simulink model "drillingRigMss"  (R2016a)
settings: Solver=VariableStepAuto  StartTime=0.0  StopTime=100  RelTol=1e-3
values from neighbouring files (symbols this model uses):
  EstimateFuelConsumption = 1    [initDrillingRigMSStoolbox.m]
  vNL0 = voltageNoQLoad*ones(engines,1)    [initDrillingRigMSStoolbox.m]
  wNL0 = 1./(1-Droop*.5)    [initDrillingRigMSStoolbox.m]
undefined symbols (not defined in the file or in its folder): magnitude, nr
undefined symbols (not defined in the file): generators
libraries: simulink x3, switchboard x1
settings Model: Creator=Elend  LastModifiedBy=torstebo
settings DataIOCC: LimitDataPoints=on  SaveFormat=Array  InspectSignalLogs=on
settings DebuggingCC: UnderspecifiedInitializationDetection=Classic  MergeDetectMultiDrivingBlocksExec=none  SolverPrmCheckMsg=warning  StateNameClashWarn=warning
settings HardwareCC: ProdBitPerPointer=32  ProdLargestAtomicFloat=None  ProdIntDivRoundTo=Undefined  ProdEndianess=Unspecified  ProdWordSize=32  ProdHWDeviceType=32-bit Generic
settings ModelReferenceCC: PropagateSignalLabelsOutOfModel=off
settings ConfigComp: CovModelRefEnable=Off

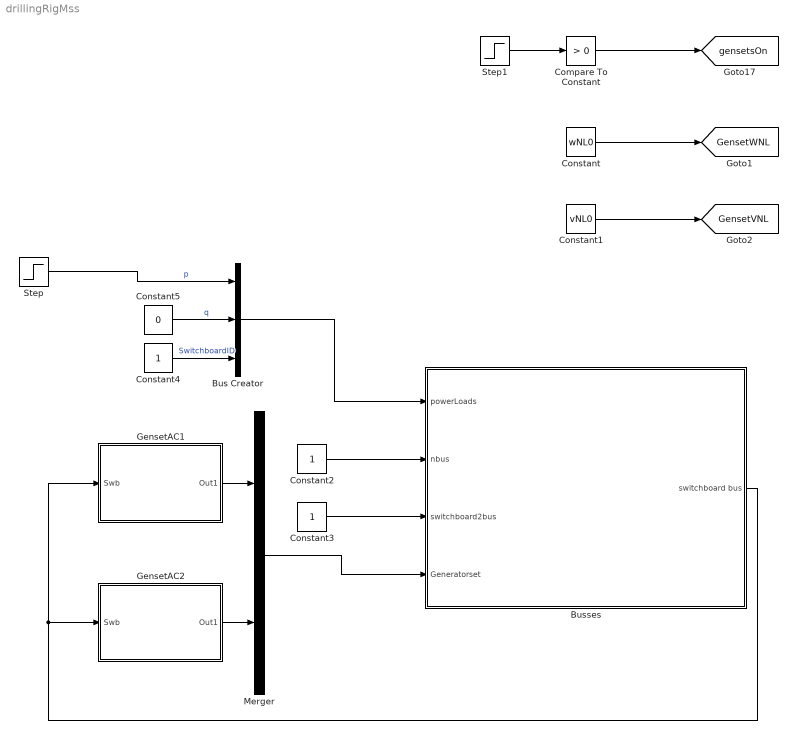
== system drillingRigMss ==
  Bus Creator : BusCreator  Inputs='p','q','SwitchboardID'  OutDataTypeStr=Bus: powerLoadsBus  NonVirtualBus=on
  Busses : Subsystem
      mask Display:
      | image(imread('figs/switchboard.jpg'))
      | port_label('input',1,'Power Loads')
      | port_label('input',2,'nbus')
      | port_label('input',3,'switchboard2bus')
      | port_label('input',4,'Generators')
      | port_label('output',1,'switchboard')
  Compare To Constant : simulink/Logic and Bit Operations/Compare To Constant  relop=>  const=0  OutDataTypeStr=boolean
  Constant : Constant  Value=wNL0
  Constant1 : Constant  Value=vNL0
  Constant2 : Constant
  Constant3 : Constant
  Constant4 : Constant
  Constant5 : Constant  Value=0
  GensetAC1 : Subsystem  Tag=GensetAC  mask{genset=generators(1), swbId=1}
      mask prompts: genset "Generator set data"; swbId "SwitchboardId"
      mask Display: image(imread('figs/generator.jpg'),'center')
  GensetAC2 : Subsystem  Tag=GensetAC  mask{genset=generators(2), swbId=1}
      mask prompts: genset "Generator set data"; swbId "SwitchboardId"
      mask Display: image(imread('figs/generator.jpg'),'center')
  Merger : Concatenate  Tag=FromGeneratorsetElectric/Merger
  Step : Step  Time=5  Before=1e6  After=2e6  SampleTime=0
  Step1 : Step  Time=50  Before=[1;1]  After=[1;0]  SampleTime=0
  tag scope: GensetVNL=global, GensetWNL=global, gensetsOn=global
  wires:
  Step1/1 -> Compare To Constant/1
  Compare To Constant/1 -> [gensetsOn]
  Constant/1 -> [GensetWNL]
  Constant1/1 -> [GensetVNL]
  Bus Creator/1 -> Busses/1(powerLoads)
  Constant3/1 -> Busses/3(switchboard2bus)
  Constant2/1 -> Busses/2(nbus)
  GensetAC2/1(Out1) -> Merger/2
  GensetAC1/1(Out1) -> Merger/1
  Merger/1 -> Busses/4(Generatorset)
  Step/1 -> Bus Creator/1  "p"
  Constant4/1 -> Bus Creator/3  "SwitchboardID"
  Constant5/1 -> Bus Creator/2  "q"
  Busses/1(switchboard bus) -> GensetAC2/1(Swb), GensetAC1/1(Swb)

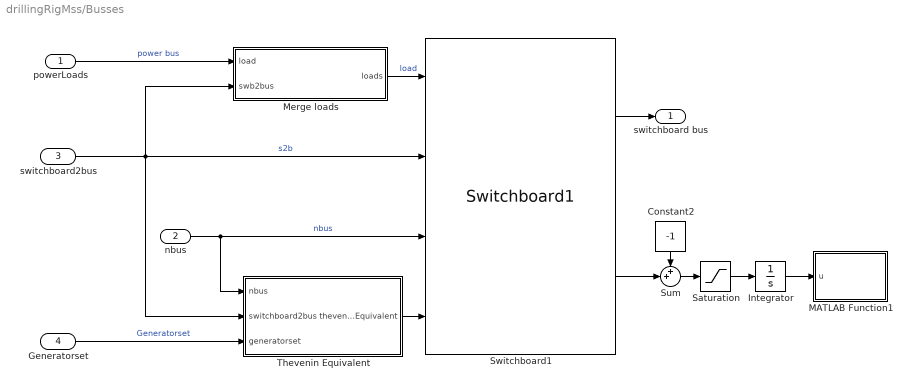
== system drillingRigMss/Busses ==
  powerLoads : Inport  OutDataTypeStr=Bus: powerLoadsBus
  nbus : Inport  Port=2
  switchboard2bus : Inport  Port=3
  Generatorset : Inport  Port=4
  Constant2 : Constant  Value=-1
  Integrator : Integrator
  MATLAB Function1 : MATLAB Function  TreatAsAtomicUnit=on
  Merge loads : MATLAB Function  TreatAsAtomicUnit=on
  Saturation : Saturate  UpperLimit=0  LowerLimit=-1
  Sum : Sum  Inputs=++|
  Switchboard1 : switchboard/Switchboard1
  Thevenin Equivalent : MATLAB Function  TreatAsAtomicUnit=on
  switchboard bus : Outport
  wires:
  Switchboard1/1 -> switchboard bus/1
  powerLoads/1 -> Merge loads/1(load)  "power bus"
  switchboard2bus/1 -> Thevenin Equivalent/2(switchboard2bus), Merge loads/2(swb2bus), Switchboard1/2  "s2b"
  Generatorset/1 -> Thevenin Equivalent/3(generatorset)  "Generatorset"
  Integrator/1 -> MATLAB Function1/1(u)
  Constant2/1 -> Sum/1
  Sum/1 -> Saturation/1
  Switchboard1/2 -> Sum/2
  nbus/1 -> Thevenin Equivalent/1(nbus), Switchboard1/3  "nbus"
  Merge loads/1(loads) -> Switchboard1/1  "load"
  Thevenin Equivalent/1(theveninEquivalent) -> Switchboard1/4
  Saturation/1 -> Integrator/1

== system drillingRigMss/GensetAC1 ==
  Swb : Inport
  Constant4 : Constant  Value=genset.ID  OutDataTypeStr=Inherit: Inherit via back propagation
  Genset : Subsystem
  Goto Tag Visibility : GotoTagVisibility  GotoTag=connected
  Selector : Selector  IndexOptions=Index vector (port)  Indices=[nr]  OutputSizes=1
  Out1 : Outport
  tag scope: connected=scoped
  wires:
  Genset/1(TheveninBus) -> Out1/1
  Constant4/1 -> Selector/2
  [gensetsOn] -> Selector/1  "Connected"
  Selector/1 -> [connected]  "Connected"
  Swb/1 -> Genset/1(Switchboard)

== system drillingRigMss/GensetAC2 ==
  Swb : Inport
  Constant4 : Constant  Value=genset.ID  OutDataTypeStr=Inherit: Inherit via back propagation
  Genset : Subsystem
  Goto Tag Visibility : GotoTagVisibility  GotoTag=connected
  Selector : Selector  IndexOptions=Index vector (port)  Indices=[nr]  OutputSizes=1
  Out1 : Outport
  tag scope: connected=scoped
  wires:
  Genset/1(TheveninBus) -> Out1/1
  Constant4/1 -> Selector/2
  [gensetsOn] -> Selector/1  "Connected"
  Selector/1 -> [connected]  "Connected"
  Swb/1 -> Genset/1(Switchboard)

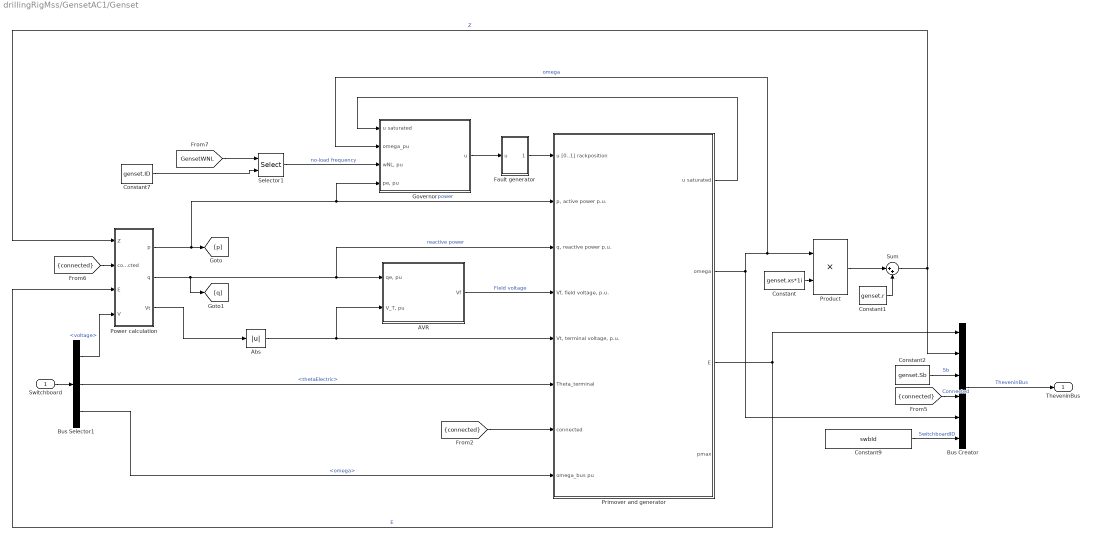
== system drillingRigMss/GensetAC1/Genset ==
  Switchboard : Inport
  AVR : Subsystem
  Abs : Abs
  Bus Creator : BusCreator  Inputs='E','Z','Sb','Connected','omega','SwitchboardID'  OutDataTypeStr=Bus: TheveninBus  NonVirtualBus=on
  Bus Selector1 : BusSelector  OutputSignals=voltage,thetaElectric,omega
  Constant : Constant  Value=genset.xs*1i
  Constant1 : Constant  Value=genset.r
  Constant2 : Constant  Value=genset.Sb
  Constant7 : Constant  Value=genset.ID  OutDataTypeStr=Inherit: Inherit via back propagation
  Constant9 : Constant  Value=swbId  OutDataTypeStr=Inherit: Inherit via back propagation
  Fault generator : Subsystem
  Governor : Subsystem
  Power calculation : MATLAB Function  TreatAsAtomicUnit=on
  Primover and generator : Subsystem
  Product : Product
  Selector1 : Selector  IndexOptions=Index vector (port)  Indices=[nr]  OutputSizes=1
  Sum : Sum  Inputs=|++
  TheveninBus : Outport
  wires:
  Constant7/1 -> Selector1/2
  Constant2/1 -> Bus Creator/3  "Sb"
  Bus Creator/1 -> TheveninBus/1  "TheveninBus"
  Sum/1 -> Bus Creator/2, Power calculation/1(Z)  "Z"
  Constant1/1 -> Sum/2
  Product/1 -> Sum/1
  Constant/1 -> Product/2
  Abs/1 -> AVR/2("V_T, pu"), Primover and generator/5("Vt, terminal voltage, p.u.")
  Power calculation/2(q) -> [q], AVR/1("qe, pu"), Primover and generator/3("q, reactive power p.u.")  "reactive power"
  Power calculation/1(p) -> [p], Governor/4("pe, pu"), Primover and generator/2("p, active power p.u.")  "power"
  [GensetWNL] -> Selector1/1
  Primover and generator/3(E) -> Bus Creator/1, Power calculation/3(E)  "E"
  Primover and generator/2(omega) -> Product/1, Governor/2(omega_pu), Bus Creator/5  "omega"
  Primover and generator/1(u saturated) -> Governor/1(u saturated)
  AVR/1(Vf) -> Primover and generator/4("Vf, field voltage, p.u.")  "Field voltage"
  Selector1/1 -> Governor/3("wNL, pu")  "no-load frequency"
  Bus Selector1/1 -> Power calculation/4(V)  "<voltage>"
  [connected] -> Primover and generator/7(connected)
  [connected] -> Power calculation/2(connected)
  [connected] -> Bus Creator/4  "Connected"
  Power calculation/3(Vt) -> Abs/1
  Bus Selector1/3 -> Primover and generator/8(omega_bus pu)  "<omega>"
  Switchboard/1 -> Bus Selector1/1
  Constant9/1 -> Bus Creator/6  "SwitchboardID"
  Bus Selector1/2 -> Primover and generator/6(Theta_terminal)  "<thetaElectric>"
  Governor/1(u) -> Fault generator/1(u)
  Fault generator/1(uOut) -> Primover and generator/1(u [0..1] rackposition)

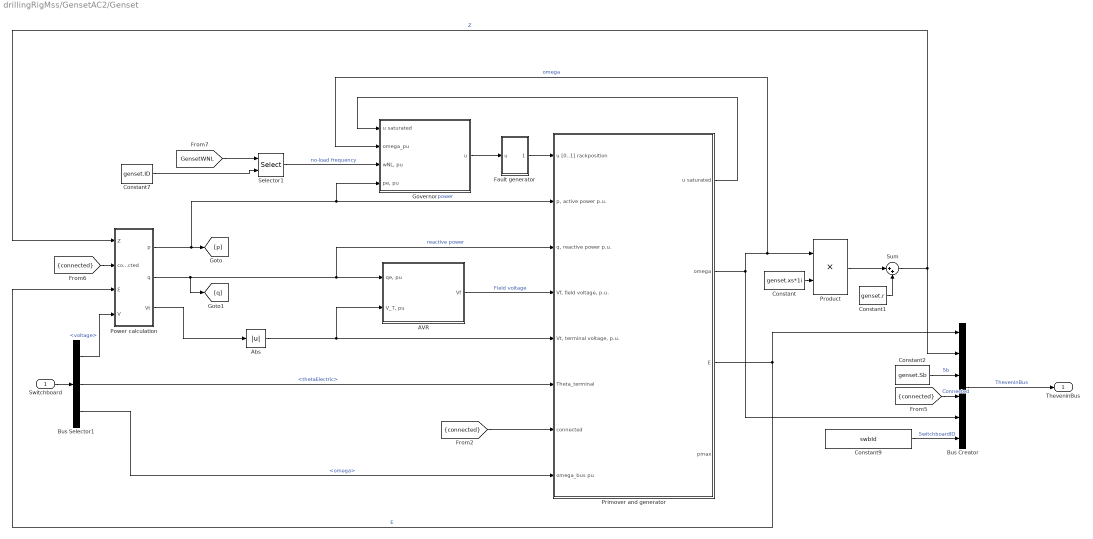
== system drillingRigMss/GensetAC2/Genset ==
  Switchboard : Inport
  AVR : Subsystem
  Abs : Abs
  Bus Creator : BusCreator  Inputs='E','Z','Sb','Connected','omega','SwitchboardID'  OutDataTypeStr=Bus: TheveninBus  NonVirtualBus=on
  Bus Selector1 : BusSelector  OutputSignals=voltage,thetaElectric,omega
  Constant : Constant  Value=genset.xs*1i
  Constant1 : Constant  Value=genset.r
  Constant2 : Constant  Value=genset.Sb
  Constant7 : Constant  Value=genset.ID  OutDataTypeStr=Inherit: Inherit via back propagation
  Constant9 : Constant  Value=swbId  OutDataTypeStr=Inherit: Inherit via back propagation
  Fault generator : Subsystem
  Governor : Subsystem
  Power calculation : MATLAB Function  TreatAsAtomicUnit=on
  Primover and generator : Subsystem
  Product : Product
  Selector1 : Selector  IndexOptions=Index vector (port)  Indices=[nr]  OutputSizes=1
  Sum : Sum  Inputs=|++
  TheveninBus : Outport
  wires:
  Constant7/1 -> Selector1/2
  Constant2/1 -> Bus Creator/3  "Sb"
  Bus Creator/1 -> TheveninBus/1  "TheveninBus"
  Sum/1 -> Bus Creator/2, Power calculation/1(Z)  "Z"
  Constant1/1 -> Sum/2
  Product/1 -> Sum/1
  Constant/1 -> Product/2
  Abs/1 -> AVR/2("V_T, pu"), Primover and generator/5("Vt, terminal voltage, p.u.")
  Power calculation/2(q) -> [q], AVR/1("qe, pu"), Primover and generator/3("q, reactive power p.u.")  "reactive power"
  Power calculation/1(p) -> [p], Governor/4("pe, pu"), Primover and generator/2("p, active power p.u.")  "power"
  [GensetWNL] -> Selector1/1
  Primover and generator/3(E) -> Bus Creator/1, Power calculation/3(E)  "E"
  Primover and generator/2(omega) -> Product/1, Governor/2(omega_pu), Bus Creator/5  "omega"
  Primover and generator/1(u saturated) -> Governor/1(u saturated)
  AVR/1(Vf) -> Primover and generator/4("Vf, field voltage, p.u.")  "Field voltage"
  Selector1/1 -> Governor/3("wNL, pu")  "no-load frequency"
  Bus Selector1/1 -> Power calculation/4(V)  "<voltage>"
  [connected] -> Primover and generator/7(connected)
  [connected] -> Power calculation/2(connected)
  [connected] -> Bus Creator/4  "Connected"
  Power calculation/3(Vt) -> Abs/1
  Bus Selector1/3 -> Primover and generator/8(omega_bus pu)  "<omega>"
  Switchboard/1 -> Bus Selector1/1
  Constant9/1 -> Bus Creator/6  "SwitchboardID"
  Bus Selector1/2 -> Primover and generator/6(Theta_terminal)  "<thetaElectric>"
  Governor/1(u) -> Fault generator/1(u)
  Fault generator/1(uOut) -> Primover and generator/1(u [0..1] rackposition)

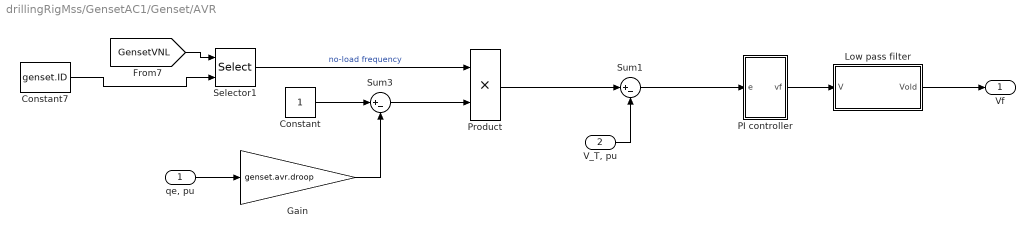
== system drillingRigMss/GensetAC1/Genset/AVR ==
  "qe, pu" : Inport
  "V_T, pu" : Inport  Port=2
  Constant : Constant
  Constant7 : Constant  Value=genset.ID  OutDataTypeStr=Inherit: Inherit via back propagation
  Gain : Gain  Gain=genset.avr.droop
  Low pass filter : Subsystem
  PI controller : Subsystem
  Product : Product  RndMeth=Zero
  Selector1 : Selector  IndexOptions=Index vector (port)  Indices=[nr]  OutputSizes=1
  Sum1 : Sum  Inputs=|+-
  Sum3 : Sum  Inputs=|+-
  Vf : Outport
  wires:
  Low pass filter/1(Vold) -> Vf/1
  Product/1 -> Sum1/1
  Sum3/1 -> Product/2
  Gain/1 -> Sum3/2
  Constant/1 -> Sum3/1
  "V_T, pu"/1 -> Sum1/2
  "qe, pu"/1 -> Gain/1
  Sum1/1 -> PI controller/1(e)
  PI controller/1(vf) -> Low pass filter/1(V)
  Constant7/1 -> Selector1/2
  [GensetVNL] -> Selector1/1
  Selector1/1 -> Product/1  "no-load frequency"

== system drillingRigMss/GensetAC1/Genset/Fault generator ==
  u : Inport
  Constant4 : Constant  Value=genset.fixThrottle
  Step : Step  Time=genset.fixThrottleTime  SampleTime=0
  Switch : Switch  Criteria=u2 > Threshold
  uOut : Outport
  wires:
  Switch/1 -> uOut/1
  u/1 -> Switch/3
  Constant4/1 -> Switch/1
  Step/1 -> Switch/2

== system drillingRigMss/GensetAC1/Genset/Governor ==
  u saturated : Inport
  omega_pu : Inport  Port=2
  "wNL, pu" : Inport  Port=3
  "pe, pu" : Inport  Port=4
  Constant : Constant
  Gain : Gain  Gain=genset.governor.droop
  PID controller : Subsystem
  Product : Product  RndMeth=Zero
  Sum : Sum  Inputs=|+-
  Sum1 : Sum  Inputs=|+-
  u : Outport
  wires:
  omega_pu/1 -> PID controller/2(omega_pu), Sum/2
  "pe, pu"/1 -> Gain/1
  u saturated/1 -> PID controller/3(u saturated)
  Sum1/1 -> Product/2
  Constant/1 -> Sum1/1
  "wNL, pu"/1 -> Product/1
  Product/1 -> Sum/1
  Sum/1 -> PID controller/1(e)
  Gain/1 -> Sum1/2
  PID controller/1(u) -> u/1  "u"

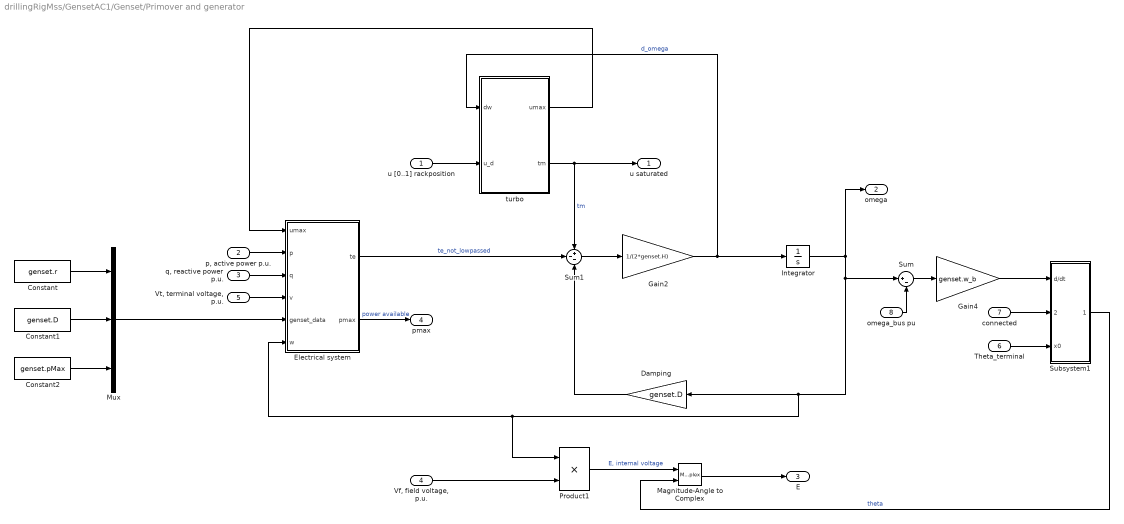
== system drillingRigMss/GensetAC1/Genset/Primover and generator ==
  u [0..1] rackposition : Inport
  "p, active power p.u." : Inport  Port=2
  "q, reactive power p.u." : Inport  Port=3
  "Vf, field voltage, p.u." : Inport  Port=4
  "Vt, terminal voltage, p.u." : Inport  Port=5
  Theta_terminal : Inport  Port=6
  connected : Inport  Port=7
  omega_bus pu : Inport  Port=8
  Constant : Constant  Value=genset.r
  Constant1 : Constant  Value=genset.D
  Constant2 : Constant  Value=genset.pMax
  Damping : Gain  Gain=genset.D
  Electrical system : MATLAB Function  TreatAsAtomicUnit=on
  Gain2 : Gain  Gain=1/(2*genset.H)
  Gain4 : Gain  Gain=genset.w_b
  Integrator : Integrator  InitialCondition=genset.omega0
  Magnitude-Angle to Complex : MagnitudeAngleToComplex
  Mux : Mux  Inputs=3
  Product1 : Product  Inputs=**  RndMeth=Zero
  Subsystem1 : Subsystem
  Sum : Sum  Inputs=|+-
  Sum1 : Sum  Inputs=+--
  turbo : Subsystem
  u saturated : Outport
  omega : Outport  Port=2
  E : Outport  Port=3
  pmax : Outport  Port=4
  wires:
  Mux/1 -> Electrical system/5(genset_data)
  Constant2/1 -> Mux/3
  Constant1/1 -> Mux/2
  Constant/1 -> Mux/1
  Magnitude-Angle to Complex/1 -> E/1
  Electrical system/2(pmax) -> pmax/1  "power available"
  turbo/1(umax) -> Electrical system/1(umax)
  Theta_terminal/1 -> Subsystem1/3(x0)
  Integrator/1 -> omega/1, Electrical system/6(w), Product1/1, Damping/1, Sum/1
  connected/1 -> Subsystem1/2(reset)
  Damping/1 -> Sum1/3
  "q, reactive power p.u."/1 -> Electrical system/3(q)
  "Vt, terminal voltage, p.u."/1 -> Electrical system/4(v)
  Electrical system/1(te) -> Sum1/2  "te_not_lowpassed"
  "p, active power p.u."/1 -> Electrical system/2(p)
  "Vf, field voltage, p.u."/1 -> Product1/2
  Gain2/1 -> Integrator/1, turbo/1(dw)  "d_omega"
  Sum1/1 -> Gain2/1
  Gain4/1 -> Subsystem1/1(d/dt)
  Subsystem1/1(Out1) -> Magnitude-Angle to Complex/2  "theta"
  Product1/1 -> Magnitude-Angle to Complex/1  "E, internal voltage"
  turbo/2(tm) -> Sum1/1, u saturated/1  "tm"
  u [0..1] rackposition/1 -> turbo/2(u_d)
  Sum/1 -> Gain4/1
  omega_bus pu/1 -> Sum/2

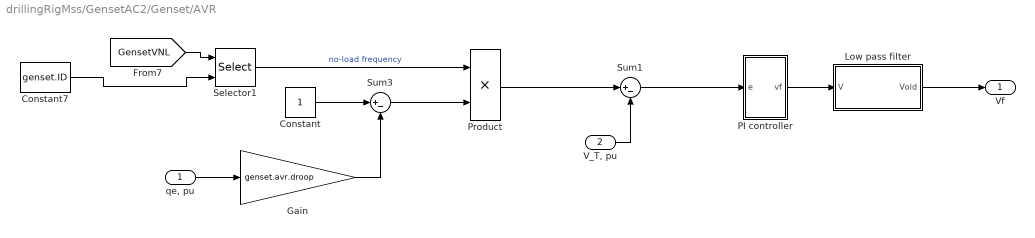
== system drillingRigMss/GensetAC2/Genset/AVR ==
  "qe, pu" : Inport
  "V_T, pu" : Inport  Port=2
  Constant : Constant
  Constant7 : Constant  Value=genset.ID  OutDataTypeStr=Inherit: Inherit via back propagation
  Gain : Gain  Gain=genset.avr.droop
  Low pass filter : Subsystem
  PI controller : Subsystem
  Product : Product  RndMeth=Zero
  Selector1 : Selector  IndexOptions=Index vector (port)  Indices=[nr]  OutputSizes=1
  Sum1 : Sum  Inputs=|+-
  Sum3 : Sum  Inputs=|+-
  Vf : Outport
  wires:
  Low pass filter/1(Vold) -> Vf/1
  Product/1 -> Sum1/1
  Sum3/1 -> Product/2
  Gain/1 -> Sum3/2
  Constant/1 -> Sum3/1
  "V_T, pu"/1 -> Sum1/2
  "qe, pu"/1 -> Gain/1
  Sum1/1 -> PI controller/1(e)
  PI controller/1(vf) -> Low pass filter/1(V)
  Constant7/1 -> Selector1/2
  [GensetVNL] -> Selector1/1
  Selector1/1 -> Product/1  "no-load frequency"

== system drillingRigMss/GensetAC2/Genset/Fault generator ==
  u : Inport
  Constant4 : Constant  Value=genset.fixThrottle
  Step : Step  Time=genset.fixThrottleTime  SampleTime=0
  Switch : Switch  Criteria=u2 > Threshold
  uOut : Outport
  wires:
  Switch/1 -> uOut/1
  u/1 -> Switch/3
  Constant4/1 -> Switch/1
  Step/1 -> Switch/2

== system drillingRigMss/GensetAC2/Genset/Governor ==
  u saturated : Inport
  omega_pu : Inport  Port=2
  "wNL, pu" : Inport  Port=3
  "pe, pu" : Inport  Port=4
  Constant : Constant
  Gain : Gain  Gain=genset.governor.droop
  PID controller : Subsystem
  Product : Product  RndMeth=Zero
  Sum : Sum  Inputs=|+-
  Sum1 : Sum  Inputs=|+-
  u : Outport
  wires:
  omega_pu/1 -> PID controller/2(omega_pu), Sum/2
  "pe, pu"/1 -> Gain/1
  u saturated/1 -> PID controller/3(u saturated)
  Sum1/1 -> Product/2
  Constant/1 -> Sum1/1
  "wNL, pu"/1 -> Product/1
  Product/1 -> Sum/1
  Sum/1 -> PID controller/1(e)
  Gain/1 -> Sum1/2
  PID controller/1(u) -> u/1  "u"

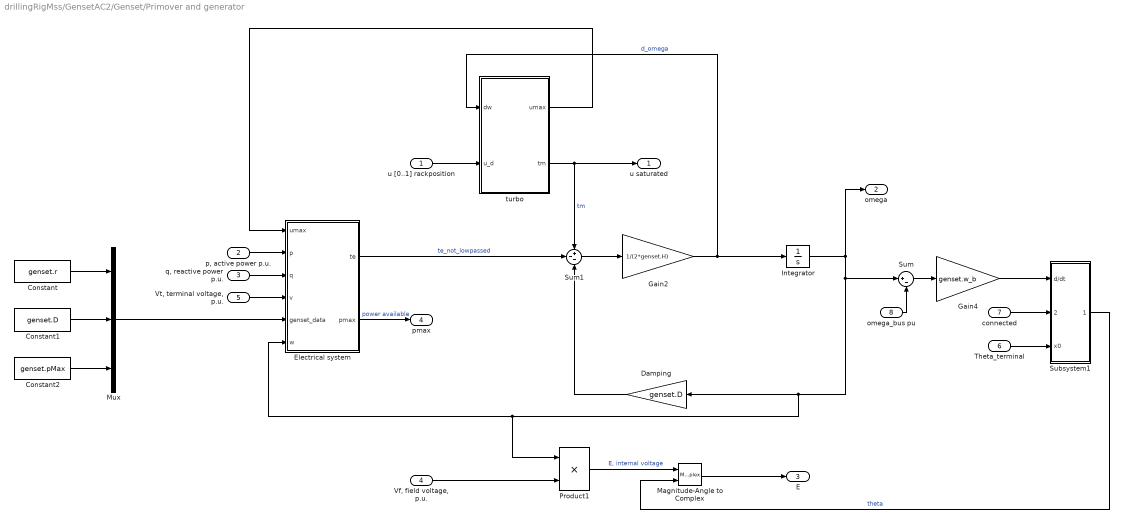
== system drillingRigMss/GensetAC2/Genset/Primover and generator ==
  u [0..1] rackposition : Inport
  "p, active power p.u." : Inport  Port=2
  "q, reactive power p.u." : Inport  Port=3
  "Vf, field voltage, p.u." : Inport  Port=4
  "Vt, terminal voltage, p.u." : Inport  Port=5
  Theta_terminal : Inport  Port=6
  connected : Inport  Port=7
  omega_bus pu : Inport  Port=8
  Constant : Constant  Value=genset.r
  Constant1 : Constant  Value=genset.D
  Constant2 : Constant  Value=genset.pMax
  Damping : Gain  Gain=genset.D
  Electrical system : MATLAB Function  TreatAsAtomicUnit=on
  Gain2 : Gain  Gain=1/(2*genset.H)
  Gain4 : Gain  Gain=genset.w_b
  Integrator : Integrator  InitialCondition=genset.omega0
  Magnitude-Angle to Complex : MagnitudeAngleToComplex
  Mux : Mux  Inputs=3
  Product1 : Product  Inputs=**  RndMeth=Zero
  Subsystem1 : Subsystem
  Sum : Sum  Inputs=|+-
  Sum1 : Sum  Inputs=+--
  turbo : Subsystem
  u saturated : Outport
  omega : Outport  Port=2
  E : Outport  Port=3
  pmax : Outport  Port=4
  wires:
  Mux/1 -> Electrical system/5(genset_data)
  Constant2/1 -> Mux/3
  Constant1/1 -> Mux/2
  Constant/1 -> Mux/1
  Magnitude-Angle to Complex/1 -> E/1
  Electrical system/2(pmax) -> pmax/1  "power available"
  turbo/1(umax) -> Electrical system/1(umax)
  Theta_terminal/1 -> Subsystem1/3(x0)
  Integrator/1 -> omega/1, Electrical system/6(w), Product1/1, Damping/1, Sum/1
  connected/1 -> Subsystem1/2(reset)
  Damping/1 -> Sum1/3
  "q, reactive power p.u."/1 -> Electrical system/3(q)
  "Vt, terminal voltage, p.u."/1 -> Electrical system/4(v)
  Electrical system/1(te) -> Sum1/2  "te_not_lowpassed"
  "p, active power p.u."/1 -> Electrical system/2(p)
  "Vf, field voltage, p.u."/1 -> Product1/2
  Gain2/1 -> Integrator/1, turbo/1(dw)  "d_omega"
  Sum1/1 -> Gain2/1
  Gain4/1 -> Subsystem1/1(d/dt)
  Subsystem1/1(Out1) -> Magnitude-Angle to Complex/2  "theta"
  Product1/1 -> Magnitude-Angle to Complex/1  "E, internal voltage"
  turbo/2(tm) -> Sum1/1, u saturated/1  "tm"
  u [0..1] rackposition/1 -> turbo/2(u_d)
  Sum/1 -> Gain4/1
  omega_bus pu/1 -> Sum/2

== system drillingRigMss/GensetAC1/Genset/AVR/Low pass filter ==
  V : Inport
  Gain : Gain  Gain=1/genset.avr.T
  Integrator : Integrator  InitialCondition=genset.avr.v0
  Sum : Sum  Inputs=|+-
  Vold : Outport
  wires:
  Gain/1 -> Integrator/1
  Sum/1 -> Gain/1
  V/1 -> Sum/1
  Integrator/1 -> Sum/2, Vold/1

== system drillingRigMss/GensetAC1/Genset/AVR/PI controller ==
  e : Inport
  Gain : Gain  Gain=genset.avr.ki
  Gain1 : Gain  Gain=genset.avr.kp
  Integrator : Integrator  DisableCoverage=on  InitialCondition=genset.avr.v0
  Saturation : Saturate  UpperLimit=genset.avr.maxFieldVoltage  LowerLimit=genset.avr.minFieldVoltage  LinearizeAsGain=off  OutMin=genset.avr.minFieldVoltage  OutMax=genset.avr.maxFieldVoltage  OutDataTypeStr=Inherit: Inherit via back propagation
  Sum : Sum  Inputs=+|+
  vf : Outport
  wires:
  Gain/1 -> Integrator/1
  Gain1/1 -> Sum/1
  Integrator/1 -> Sum/2
  e/1 -> Gain1/1, Gain/1
  Sum/1 -> Saturation/1
  Saturation/1 -> vf/1

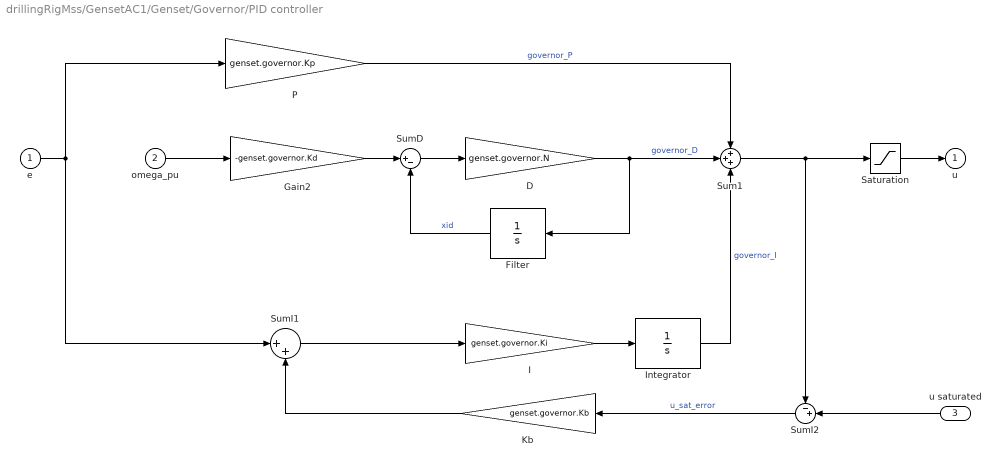
== system drillingRigMss/GensetAC1/Genset/Governor/PID controller ==
  e : Inport  PortDimensions=1
  omega_pu : Inport  Port=2  PortDimensions=1
  u saturated : Inport  Port=3  PortDimensions=1
  D : Gain  DisableCoverage=on  Gain=genset.governor.N
  Filter : Integrator  DisableCoverage=on  InitialCondition=-genset.omega0*genset.governor.Kd
  Gain2 : Gain  Gain=-genset.governor.Kd
  I : Gain  Gain=genset.governor.Ki
  Integrator : Integrator  DisableCoverage=on  InitialCondition=genset.u0
  Kb : Gain  DisableCoverage=on  Gain=genset.governor.Kb  ParamDataTypeStr=Inherit: Inherit from 'Gain'
  P : Gain  Gain=genset.governor.Kp
  Saturation : Saturate  UpperLimit=genset.uMax  LowerLimit=genset.uMin  LinearizeAsGain=off  OutMin=genset.uMin  OutMax=genset.uMax  OutDataTypeStr=Inherit: Inherit via back propagation
  Sum1 : Sum  Inputs=+++
  SumD : Sum  DisableCoverage=on  Inputs=|+-
  SumI1 : Sum  DisableCoverage=on  Inputs=|++
  SumI2 : Sum  DisableCoverage=on  Inputs=-+|
  u : Outport  PortDimensions=1  InitialOutput=0
  wires:
  I/1 -> Integrator/1
  SumI1/1 -> I/1
  u saturated/1 -> SumI2/2
  Kb/1 -> SumI1/2
  SumI2/1 -> Kb/1  "u_sat_error"
  Sum1/1 -> SumI2/1, Saturation/1
  Gain2/1 -> SumD/1
  SumD/1 -> D/1
  Filter/1 -> SumD/2  "xid"
  Saturation/1 -> u/1
  P/1 -> Sum1/1  "governor_P"
  e/1 -> SumI1/1, P/1
  omega_pu/1 -> Gain2/1
  D/1 -> Filter/1, Sum1/2  "governor_D"
  Integrator/1 -> Sum1/3  "governor_I"

== system drillingRigMss/GensetAC1/Genset/Primover and generator/Subsystem1 ==
  d/dt : Inport
  reset : Inport  Port=2
  x0 : Inport  Port=3
  Gain : Gain  Gain=1000
  Integrator : Integrator  InitialCondition=genset.theta0
  MATLAB Function : MATLAB Function  TreatAsAtomicUnit=on
  Sum : Sum  Inputs=-|+
  Switch : Switch  Threshold=1
  Out1 : Outport
  wires:
  Switch/1 -> Integrator/1
  d/dt/1 -> Switch/1
  MATLAB Function/1(y) -> Gain/1
  Gain/1 -> Switch/3
  Sum/1 -> MATLAB Function/1(u)
  x0/1 -> Sum/2
  reset/1 -> Switch/2
  Integrator/1 -> Sum/1, Out1/1

== system drillingRigMss/GensetAC1/Genset/Primover and generator/turbo ==
  dw : Inport
  u_d : Inport  Port=2
  Constant : Constant  Value=EstimateFuelConsumption
  Subsystem : Subsystem
  dead-band rate limiter : Subsystem  mask(Rate limiter for diesel engines){umax=genset.uMax, umin=genset.uMin}
      mask prompts: umax "Static maximum torque"; umin "Static minimum torque"
      mask help:
      | Allows the input to change within a delta limit, however if the input
      | changes more than this range will the input be saturated by a rate limiter.
  umax : Outport
  tm : Outport  Port=2
  wires:
  dead-band rate limiter/1(u_max) -> umax/1
  u_d/1 -> dead-band rate limiter/1(u_d)
  dead-band rate limiter/2(u_saturated) -> Subsystem/2(tm), tm/1  "tm"
  dw/1 -> Subsystem/1(dw)
  Constant/1 -> Subsystem/Enable

== system drillingRigMss/GensetAC2/Genset/AVR/Low pass filter ==
  V : Inport
  Gain : Gain  Gain=1/genset.avr.T
  Integrator : Integrator  InitialCondition=genset.avr.v0
  Sum : Sum  Inputs=|+-
  Vold : Outport
  wires:
  Gain/1 -> Integrator/1
  Sum/1 -> Gain/1
  V/1 -> Sum/1
  Integrator/1 -> Sum/2, Vold/1

== system drillingRigMss/GensetAC2/Genset/AVR/PI controller ==
  e : Inport
  Gain : Gain  Gain=genset.avr.ki
  Gain1 : Gain  Gain=genset.avr.kp
  Integrator : Integrator  DisableCoverage=on  InitialCondition=genset.avr.v0
  Saturation : Saturate  UpperLimit=genset.avr.maxFieldVoltage  LowerLimit=genset.avr.minFieldVoltage  LinearizeAsGain=off  OutMin=genset.avr.minFieldVoltage  OutMax=genset.avr.maxFieldVoltage  OutDataTypeStr=Inherit: Inherit via back propagation
  Sum : Sum  Inputs=+|+
  vf : Outport
  wires:
  Gain/1 -> Integrator/1
  Gain1/1 -> Sum/1
  Integrator/1 -> Sum/2
  e/1 -> Gain1/1, Gain/1
  Sum/1 -> Saturation/1
  Saturation/1 -> vf/1

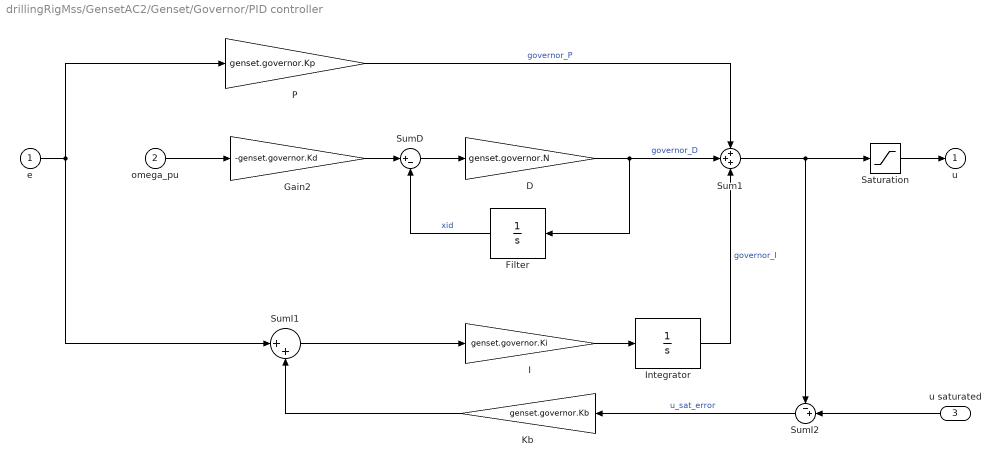
== system drillingRigMss/GensetAC2/Genset/Governor/PID controller ==
  e : Inport  PortDimensions=1
  omega_pu : Inport  Port=2  PortDimensions=1
  u saturated : Inport  Port=3  PortDimensions=1
  D : Gain  DisableCoverage=on  Gain=genset.governor.N
  Filter : Integrator  DisableCoverage=on  InitialCondition=-genset.omega0*genset.governor.Kd
  Gain2 : Gain  Gain=-genset.governor.Kd
  I : Gain  Gain=genset.governor.Ki
  Integrator : Integrator  DisableCoverage=on  InitialCondition=genset.u0
  Kb : Gain  DisableCoverage=on  Gain=genset.governor.Kb  ParamDataTypeStr=Inherit: Inherit from 'Gain'
  P : Gain  Gain=genset.governor.Kp
  Saturation : Saturate  UpperLimit=genset.uMax  LowerLimit=genset.uMin  LinearizeAsGain=off  OutMin=genset.uMin  OutMax=genset.uMax  OutDataTypeStr=Inherit: Inherit via back propagation
  Sum1 : Sum  Inputs=+++
  SumD : Sum  DisableCoverage=on  Inputs=|+-
  SumI1 : Sum  DisableCoverage=on  Inputs=|++
  SumI2 : Sum  DisableCoverage=on  Inputs=-+|
  u : Outport  PortDimensions=1  InitialOutput=0
  wires:
  I/1 -> Integrator/1
  SumI1/1 -> I/1
  u saturated/1 -> SumI2/2
  Kb/1 -> SumI1/2
  SumI2/1 -> Kb/1  "u_sat_error"
  Sum1/1 -> SumI2/1, Saturation/1
  Gain2/1 -> SumD/1
  SumD/1 -> D/1
  Filter/1 -> SumD/2  "xid"
  Saturation/1 -> u/1
  P/1 -> Sum1/1  "governor_P"
  e/1 -> SumI1/1, P/1
  omega_pu/1 -> Gain2/1
  D/1 -> Filter/1, Sum1/2  "governor_D"
  Integrator/1 -> Sum1/3  "governor_I"

== system drillingRigMss/GensetAC2/Genset/Primover and generator/Subsystem1 ==
  d/dt : Inport
  reset : Inport  Port=2
  x0 : Inport  Port=3
  Gain : Gain  Gain=1000
  Integrator : Integrator  InitialCondition=genset.theta0
  MATLAB Function : MATLAB Function  TreatAsAtomicUnit=on
  Sum : Sum  Inputs=-|+
  Switch : Switch  Threshold=1
  Out1 : Outport
  wires:
  Switch/1 -> Integrator/1
  d/dt/1 -> Switch/1
  MATLAB Function/1(y) -> Gain/1
  Gain/1 -> Switch/3
  Sum/1 -> MATLAB Function/1(u)
  x0/1 -> Sum/2
  reset/1 -> Switch/2
  Integrator/1 -> Sum/1, Out1/1

== system drillingRigMss/GensetAC2/Genset/Primover and generator/turbo ==
  dw : Inport
  u_d : Inport  Port=2
  Constant : Constant  Value=EstimateFuelConsumption
  Subsystem : Subsystem
  dead-band rate limiter : Subsystem  mask(Rate limiter for diesel engines){umax=genset.uMax, umin=genset.uMin}
      mask prompts: umax "Static maximum torque"; umin "Static minimum torque"
      mask help:
      | Allows the input to change within a delta limit, however if the input
      | changes more than this range will the input be saturated by a rate limiter.
  umax : Outport
  tm : Outport  Port=2
  wires:
  dead-band rate limiter/1(u_max) -> umax/1
  u_d/1 -> dead-band rate limiter/1(u_d)
  dead-band rate limiter/2(u_saturated) -> Subsystem/2(tm), tm/1  "tm"
  dw/1 -> Subsystem/1(dw)
  Constant/1 -> Subsystem/Enable

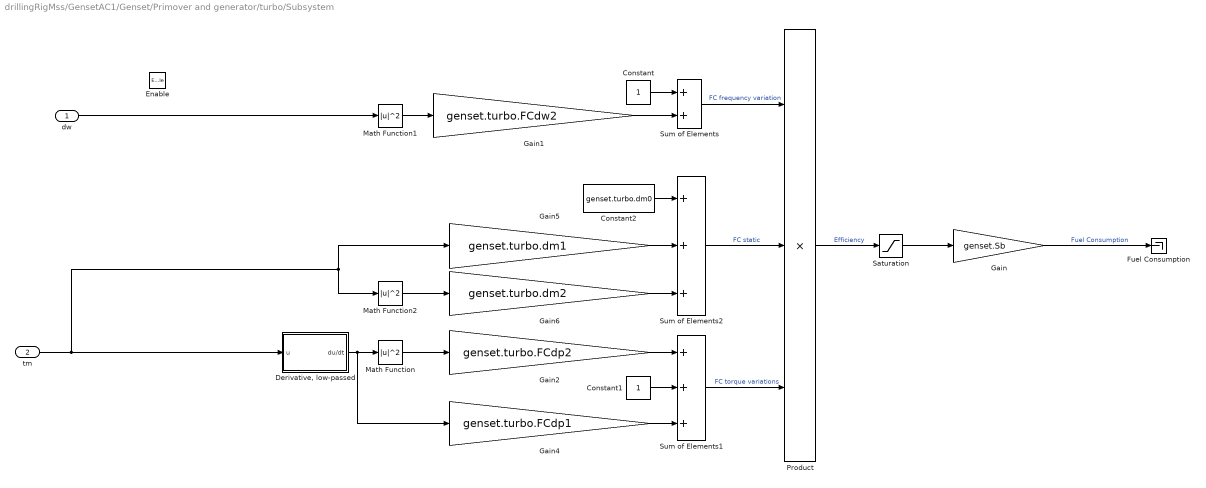
== system drillingRigMss/GensetAC1/Genset/Primover and generator/turbo/Subsystem ==
  dw : Inport
  tm : Inport  Port=2
  Enable : EnablePort
  Constant : Constant
  Constant1 : Constant
  Constant2 : Constant  Value=genset.turbo.dm0
  "Derivative, low-passed" : Subsystem
      settings: MinAlgLoopOccurrences=on
  Fuel Consumption : Terminator
  Gain : Gain  Gain=genset.Sb
  Gain1 : Gain  Gain=genset.turbo.FCdw2
  Gain2 : Gain  Gain=genset.turbo.FCdp2
  Gain4 : Gain  Gain=genset.turbo.FCdp1
  Gain5 : Gain  Gain=genset.turbo.dm1
  Gain6 : Gain  Gain=genset.turbo.dm2
  Math Function : Math  Operator=magnitude^2  SaturateOnIntegerOverflow=on
  Math Function1 : Math  Operator=magnitude^2  SaturateOnIntegerOverflow=on
  Math Function2 : Math  Operator=magnitude^2  SaturateOnIntegerOverflow=on
  Product : Product  Inputs=3  RndMeth=Zero
  Saturation : Saturate  UpperLimit=genset.turbo.FCmax  LowerLimit=0
  Sum of Elements : Sum
  Sum of Elements1 : Sum  Inputs=+++
  Sum of Elements2 : Sum  Inputs=+++
  wires:
  tm/1 -> Math Function2/1, Gain5/1, "Derivative, low-passed"/1(u)
  dw/1 -> Math Function1/1
  "Derivative, low-passed"/1(du/dt) -> Gain4/1, Math Function/1
  Math Function1/1 -> Gain1/1
  Math Function/1 -> Gain2/1
  Gain1/1 -> Sum of Elements/2
  Constant/1 -> Sum of Elements/1
  Gain2/1 -> Sum of Elements1/1
  Gain4/1 -> Sum of Elements1/3
  Constant1/1 -> Sum of Elements1/2
  Gain6/1 -> Sum of Elements2/3
  Gain5/1 -> Sum of Elements2/2
  Constant2/1 -> Sum of Elements2/1
  Math Function2/1 -> Gain6/1
  Sum of Elements1/1 -> Product/3  "FC torque variations"
  Sum of Elements2/1 -> Product/2  "FC static"
  Sum of Elements/1 -> Product/1  "FC frequency variation"
  Product/1 -> Saturation/1  "Efficiency"
  Saturation/1 -> Gain/1
  Gain/1 -> Fuel Consumption/1  "Fuel Consumption"

== system drillingRigMss/GensetAC1/Genset/Primover and generator/turbo/dead-band rate limiter ==
  u_d : Inport
  Constant : Constant  Value=umin
  Constant1 : Constant  Value=genset.governor.deltaU
  Delta : MATLAB Function  Commented=on  TreatAsAtomicUnit=on
  Gain : Gain  Gain=10
  Integrator : Integrator  InitialCondition=umax  LimitOutput=on  LowerSaturationLimit=umin
  Saturation : Saturate  UpperLimit=genset.governor.rampMax  LowerLimit=-.2
  Saturation Dynamic : simulink/Discontinuities/Saturation Dynamic  OutMin=[]  OutMax=[]  OutDataTypeStr=Inherit: Same as second input  OutDataType=fixdt(1, 16)  OutScaling=2^-10  DoSatur=off
  Sum : Sum  Inputs=|+++
  Sum1 : Sum  Inputs=-+|
  u_max : Outport
  u_saturated : Outport  Port=2
  wires:
  Constant1/1 -> Sum/3
  Delta/1(delta) -> Sum/2
  Saturation Dynamic/1 -> u_saturated/1, Sum/1, Delta/1(p)  "usat"
  Saturation/1 -> Integrator/1
  Integrator/1 -> Saturation Dynamic/1, Sum1/1, u_max/1  "umax"
  u_d/1 -> Saturation Dynamic/2  "ud"
  Constant/1 -> Saturation Dynamic/3
  Sum/1 -> Sum1/2  "u+delta"
  Sum1/1 -> Gain/1
  Gain/1 -> Saturation/1

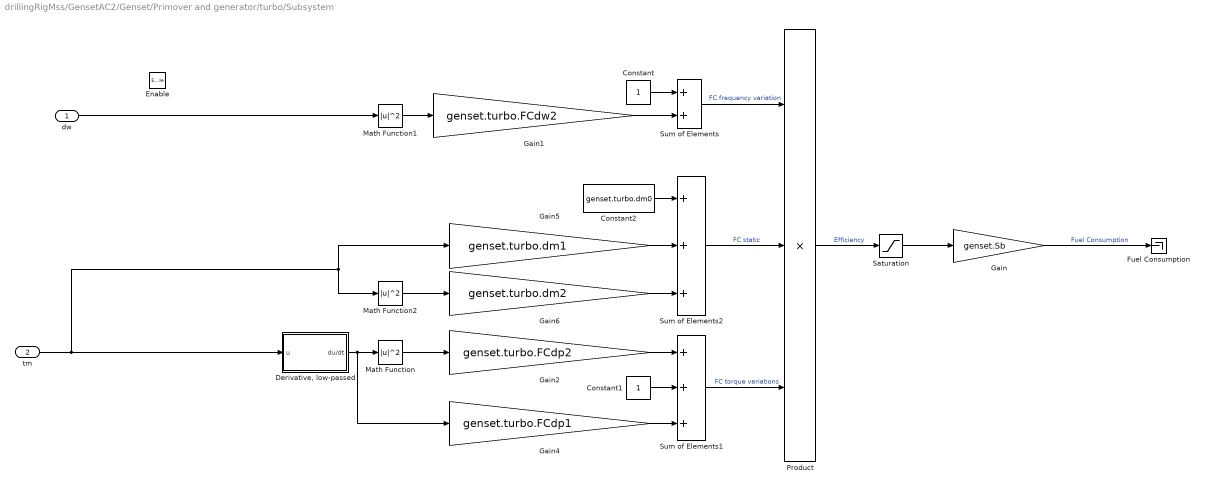
== system drillingRigMss/GensetAC2/Genset/Primover and generator/turbo/Subsystem ==
  dw : Inport
  tm : Inport  Port=2
  Enable : EnablePort
  Constant : Constant
  Constant1 : Constant
  Constant2 : Constant  Value=genset.turbo.dm0
  "Derivative, low-passed" : Subsystem
      settings: MinAlgLoopOccurrences=on
  Fuel Consumption : Terminator
  Gain : Gain  Gain=genset.Sb
  Gain1 : Gain  Gain=genset.turbo.FCdw2
  Gain2 : Gain  Gain=genset.turbo.FCdp2
  Gain4 : Gain  Gain=genset.turbo.FCdp1
  Gain5 : Gain  Gain=genset.turbo.dm1
  Gain6 : Gain  Gain=genset.turbo.dm2
  Math Function : Math  Operator=magnitude^2  SaturateOnIntegerOverflow=on
  Math Function1 : Math  Operator=magnitude^2  SaturateOnIntegerOverflow=on
  Math Function2 : Math  Operator=magnitude^2  SaturateOnIntegerOverflow=on
  Product : Product  Inputs=3  RndMeth=Zero
  Saturation : Saturate  UpperLimit=genset.turbo.FCmax  LowerLimit=0
  Sum of Elements : Sum
  Sum of Elements1 : Sum  Inputs=+++
  Sum of Elements2 : Sum  Inputs=+++
  wires:
  tm/1 -> Math Function2/1, Gain5/1, "Derivative, low-passed"/1(u)
  dw/1 -> Math Function1/1
  "Derivative, low-passed"/1(du/dt) -> Gain4/1, Math Function/1
  Math Function1/1 -> Gain1/1
  Math Function/1 -> Gain2/1
  Gain1/1 -> Sum of Elements/2
  Constant/1 -> Sum of Elements/1
  Gain2/1 -> Sum of Elements1/1
  Gain4/1 -> Sum of Elements1/3
  Constant1/1 -> Sum of Elements1/2
  Gain6/1 -> Sum of Elements2/3
  Gain5/1 -> Sum of Elements2/2
  Constant2/1 -> Sum of Elements2/1
  Math Function2/1 -> Gain6/1
  Sum of Elements1/1 -> Product/3  "FC torque variations"
  Sum of Elements2/1 -> Product/2  "FC static"
  Sum of Elements/1 -> Product/1  "FC frequency variation"
  Product/1 -> Saturation/1  "Efficiency"
  Saturation/1 -> Gain/1
  Gain/1 -> Fuel Consumption/1  "Fuel Consumption"

== system drillingRigMss/GensetAC2/Genset/Primover and generator/turbo/dead-band rate limiter ==
  u_d : Inport
  Constant : Constant  Value=umin
  Constant1 : Constant  Value=genset.governor.deltaU
  Delta : MATLAB Function  Commented=on  TreatAsAtomicUnit=on
  Gain : Gain  Gain=10
  Integrator : Integrator  InitialCondition=umax  LimitOutput=on  LowerSaturationLimit=umin
  Saturation : Saturate  UpperLimit=genset.governor.rampMax  LowerLimit=-.2
  Saturation Dynamic : simulink/Discontinuities/Saturation Dynamic  OutMin=[]  OutMax=[]  OutDataTypeStr=Inherit: Same as second input  OutDataType=fixdt(1, 16)  OutScaling=2^-10  DoSatur=off
  Sum : Sum  Inputs=|+++
  Sum1 : Sum  Inputs=-+|
  u_max : Outport
  u_saturated : Outport  Port=2
  wires:
  Constant1/1 -> Sum/3
  Delta/1(delta) -> Sum/2
  Saturation Dynamic/1 -> u_saturated/1, Sum/1, Delta/1(p)  "usat"
  Saturation/1 -> Integrator/1
  Integrator/1 -> Saturation Dynamic/1, Sum1/1, u_max/1  "umax"
  u_d/1 -> Saturation Dynamic/2  "ud"
  Constant/1 -> Saturation Dynamic/3
  Sum/1 -> Sum1/2  "u+delta"
  Sum1/1 -> Gain/1
  Gain/1 -> Saturation/1

== system drillingRigMss/GensetAC1/Genset/Primover and generator/turbo/Subsystem/Derivative, low-passed ==
  u : Inport
  Gain : Gain  Gain=10
  Integrator : Integrator  InitialCondition=genset.u0
  Sum : Sum  Inputs=|+-
  du/dt : Outport
  wires:
  u/1 -> Sum/1
  Gain/1 -> Integrator/1, du/dt/1
  Integrator/1 -> Sum/2
  Sum/1 -> Gain/1

== system drillingRigMss/GensetAC2/Genset/Primover and generator/turbo/Subsystem/Derivative, low-passed ==
  u : Inport
  Gain : Gain  Gain=10
  Integrator : Integrator  InitialCondition=genset.u0
  Sum : Sum  Inputs=|+-
  du/dt : Outport
  wires:
  u/1 -> Sum/1
  Gain/1 -> Integrator/1, du/dt/1
  Integrator/1 -> Sum/2
  Sum/1 -> Gain/1

== matlab function drillingRigMss/Busses/MATLAB Function1 ==
  data: u input
function stopper(u)
%#codegen
if ( u < -1)
    error('Bus voltage calculations have been invalid for 1 second, stopping stimulation');
end

== matlab function drillingRigMss/GensetAC1/Genset/Power calculation ==
  data: Z input; connected input; p output; E input; V input; q output; Vt output
function [p,q,Vt] = power(Z,connected,E,V)
%#codegen
if (connected)
Vt = V;
V = V/sqrt(3);
s = 3*V.*conj((E-V)./Z);
p = real(s);
q = imag(s);

else
p = 0;
q = 0;
Vt =E*sqrt(3);
end

== matlab function drillingRigMss/GensetAC1/Genset/Primover and generator/Electrical system ==
  data: umax input; p input size=1; q input; v input; genset_data input; te output; w input; pmax output size=1
function [te,pmax] = fcn(umax,p,q,v,genset_data,w)
r     = genset_data(1);
D     = genset_data(2);
p_max = genset_data(3);

te = (p+r*(p^2+q^2)/v^2)/w;
pmax = min((v/(1+r))*(-D*w^2+umax*w-r*q^2/v),p_max);

== matlab function drillingRigMss/Busses/Merge loads ==
  data: load input; loads output Bus: powerLoadsBus; swb2bus input
function loads  = mergeloads(load,swb2bus)
%#codegen
loads = repmat( struct( 'p',0,'q',0,'SwitchboardID',0),length(swb2bus),1);
for i = 1:length(load)
    bus = swb2bus(load(i).SwitchboardID);
    loads(bus).p = loads(bus).p+ load(i).p;
    loads(bus).q = loads(bus).q+ load(i).q;
end
for i = 1:length(swb2bus)
    loads(i).SwitchboardID = i;
end

== matlab function drillingRigMss/GensetAC1/Genset/Primover and generator/Subsystem1/MATLAB Function ==
  data: u input; y output
function y = fcn(u)
%#codegen

y = anglemap(u);

== matlab function drillingRigMss/GensetAC1/Genset/Primover and generator/turbo/dead-band rate limiter/Delta ==
  data: p input; delta output
function delta = fcn(p)
%#codegen
if p<.33
    delta = .33-.303*p;
elseif p<.56
    delta = .3-.217*p;
elseif p<.74
    delta = -.068+.444*p;
else
    delta = .26;
end

== matlab function drillingRigMss/GensetAC2/Genset/Power calculation ==
  data: Z input; connected input; p output; E input; V input; q output; Vt output
function [p,q,Vt] = power(Z,connected,E,V)
%#codegen
if (connected)
Vt = V;
V = V/sqrt(3);
s = 3*V.*conj((E-V)./Z);
p = real(s);
q = imag(s);

else
p = 0;
q = 0;
Vt =E*sqrt(3);
end

== matlab function drillingRigMss/GensetAC2/Genset/Primover and generator/Electrical system ==
  data: umax input; p input size=1; q input; v input; genset_data input; te output; w input; pmax output size=1
function [te,pmax] = fcn(umax,p,q,v,genset_data,w)
r     = genset_data(1);
D     = genset_data(2);
p_max = genset_data(3);

te = (p+r*(p^2+q^2)/v^2)/w;
pmax = min((v/(1+r))*(-D*w^2+umax*w-r*q^2/v),p_max);

== matlab function drillingRigMss/Busses/Thevenin Equivalent ==
  data: nbus input; switchboard2bus input; generatorset input; theveninEquivalent output Bus: TheveninBus
function theveninEquivalent  = mergeGenerators(nbus,switchboard2bus,generatorset)
%#codegen
nSwitchboards = length(switchboard2bus);
assert(nbus<=nSwitchboards);
nGeneratorset = length(generatorset);
E = complex(zeros(nGeneratorset,1));
Z = complex(zeros(nGeneratorset,1));
Sb = zeros(nGeneratorset,1);
Connected = zeros(nGeneratorset,1);
omega = zeros(nGeneratorset,1);
genset2swb = zeros(nGeneratorset,1);
for i = 1:nGeneratorset
    E(i) = generatorset(i).E;
    Z(i) = generatorset(i).Z;
    Sb(i) = generatorset(i).Sb;
    Connected(i) = generatorset(i).Connected;
    omega(i) = generatorset(i).omega;
    genset2swb(i) = generatorset(i).SwitchboardID;
end   

theveninEquivalent = repmat( struct( 'E',1j,'Z',1j,'Sb',0,'Connected',true,'omega',0,'SwitchboardID',0),nSwitchboards);
for bus = 1:nbus
    %Find gensets connected to bus
    m = 0;  
    for i = 1:nGeneratorset
        if (switchboard2bus(genset2swb(i))==bus && Connected(i))
            m = m + 1;
        end
    end
    assert(m <= nGeneratorset);
    gensets = zeros(1,m);
    m = 0;    
    for i = 1:nGeneratorset
        if (switchboard2bus(genset2swb(i))==bus && Connected(i))
            m = m + 1;
            gensets(m) = i;
        end
    end
    [ et, zt, Sb_bus, ~, omegaAvgBus ] = TheveninEquivalent( E(gensets), Z(gensets), Sb(gensets), Connected(gensets), omega(gensets) );
    theveninEquivalent(bus).E = et;
    theveninEquivalent(bus).Z = zt;
    theveninEquivalent(bus).Sb = Sb_bus;
    theveninEquivalent(bus).Connected = true;
    theveninEquivalent(bus).omega = omegaAvgBus;
    theveninEquivalent(bus).SwitchboardID = bus;
end

== matlab function drillingRigMss/GensetAC2/Genset/Primover and generator/Subsystem1/MATLAB Function ==
  data: u input; y output
function y = fcn(u)
%#codegen

y = anglemap(u);

== matlab function drillingRigMss/GensetAC2/Genset/Primover and generator/turbo/dead-band rate limiter/Delta ==
  data: p input; delta output
function delta = fcn(p)
%#codegen
if p<.33
    delta = .33-.303*p;
elseif p<.56
    delta = .3-.217*p;
elseif p<.74
    delta = -.068+.444*p;
else
    delta = .26;
end
